simulink model "motion_with_control"  (R2025a)
settings: Solver=FixedStepDiscrete  StartTime=0.0  StopTime=inf  FixedStep=0.01  RelTol=1e-3  EnableMultiTasking=on
PreLoadFcn:
  | frs = FrankaRobotSettings;
libraries: franka_simulink x3
settings Model: SimulationMode=external  ExtModeTrigDuration=10000  Creator=vasi_ko  LastModifiedBy=kvasios
settings SolverCC: ConcurrentTasks=on  AlgebraicLoopSolver=TrustRegion  InsertRTBMode=Never (minimum delay)
settings DataIOCC: LimitDataPoints=on  SaveFormat=Array  ReturnWorkspaceOutputs=off
settings OptimizationCC: DefaultParameterBehavior=Inlined  EnhancedBackFolding=on  PassReuseOutputArgsThreshold=0.0  MaxStackSize=200000  OptimizeBlockOrder=speed  DifferentSizesBufferReuse=on  OptimizationCustomize=off
settings DebuggingCC: SolverPrmCheckMsg=warning  ParameterTunabilityLossMsg=error  UnconnectedInputMsg=warning  UnconnectedOutputMsg=warning  UnconnectedLineMsg=warning  SFUnexpectedBacktrackingDiag=warning  SFNoUnconditionalDefaultTransitionDiag=warning  SFExecutionAtInitializationDiag=none  ArithmeticOperatorsInVariantConditions=warning
settings HardwareCC: ProdBitPerLong=64.0  ProdHWDeviceType=Intel->x86-64 (Linux 64)
settings ModelReferenceCC: EnableRefExpFcnMdlSchedulingChecks=on  PropagateSignalLabelsOutOfModel=off
settings SFSimCC: SimUseLocalCustomCode=off  MATLABDynamicMemAlloc=off  CustomCodeUndefinedFunction=UseInterfaceOnly  SimTargetLang=C++  SimDLTargetLibrary=mkl-dnn
settings RTWCC: HardwareBoard=Generic Linux AMD64 Board  RTWVerbose=off  RTWUseLocalCustomCode=off  BuildConfiguration=Faster Runs  TargetLang=C++  GPUComputeCapability=3.5  DLArmComputeVersion=19.05
settings CodeAppCC: ForceParamTrailComments=on  OperatorAnnotations=on
settings GRTTargetCC: ExtModeStaticAlloc=on  ExtModeMexFile=ext_xcp  ExtModeIntrfLevel=Level2 - Open  MultiInstanceErrorCode=Warning  TargetLangStandard=C++14 (ISO)
settings ConfigComp: CovMetricSettings=dw  CovSaveCumulativeToWorkspaceVar=on  CovSaveSingleToWorkspaceVar=on  CovExternalEMLEnable=off  CovSFcnEnable=off

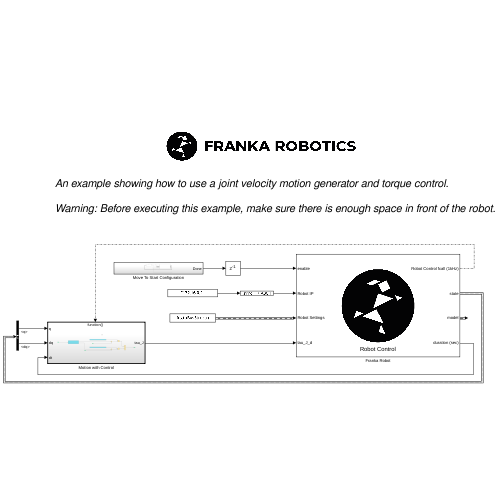
[thumbnail: Simulink's stored preview of the top-level diagram]
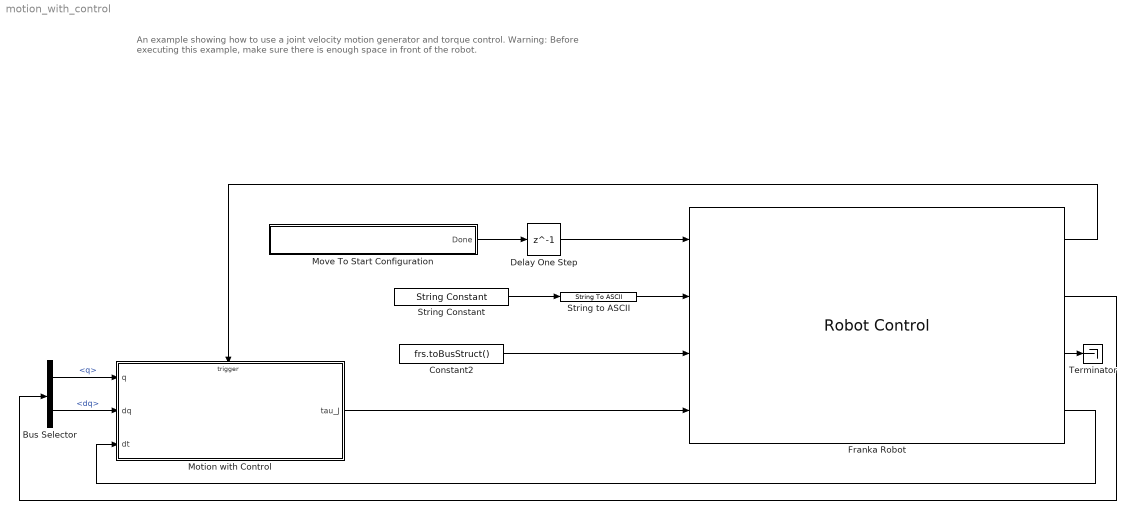
== system motion_with_control ==
  note: An example showing how to use a joint velocity motion generator and torque control.
      |
      | Warning: Before executing this example, make sure there is enough space in front of the robot.
  Bus Selector : BusSelector  OutputSignals=q,dq
  Constant2 : Constant  Value=frs.toBusStruct()  OutDataTypeStr=Bus: FrankaRobotSettingsBus
  Delay One Step : Delay  DelayLength=1
  Franka Robot : franka_simulink/Robot Control  control_mode=Torques
      settings: SourceProductName=Franka Robotics Simulink Support Package
  Motion with Control : Subsystem
      settings: RTWSystemCode=Nonreusable function
  Move To Start Configuration : Subsystem
  String Constant : StringConstant  String="\"172.16.0.2\""
  String to ASCII : StringToASCII  OutputVectorSize=16
  Terminator : Terminator
  wires:
  String to ASCII/1 -> Franka Robot/2
  String Constant/1 -> String to ASCII/1
  Franka Robot/1 -> Motion with Control/Trigger
  Franka Robot/2 -> Bus Selector/1
  Bus Selector/1 -> Motion with Control/1(q)  "<q>"
  Bus Selector/2 -> Motion with Control/2(dq)  "<dq>"
  Franka Robot/4 -> Motion with Control/3(dt)
  Franka Robot/3 -> Terminator/1
  Constant2/1 -> Franka Robot/3
  Motion with Control/1(tau_J) -> Franka Robot/4
  Delay One Step/1 -> Franka Robot/1
  Move To Start Configuration/1(Done) -> Delay One Step/1

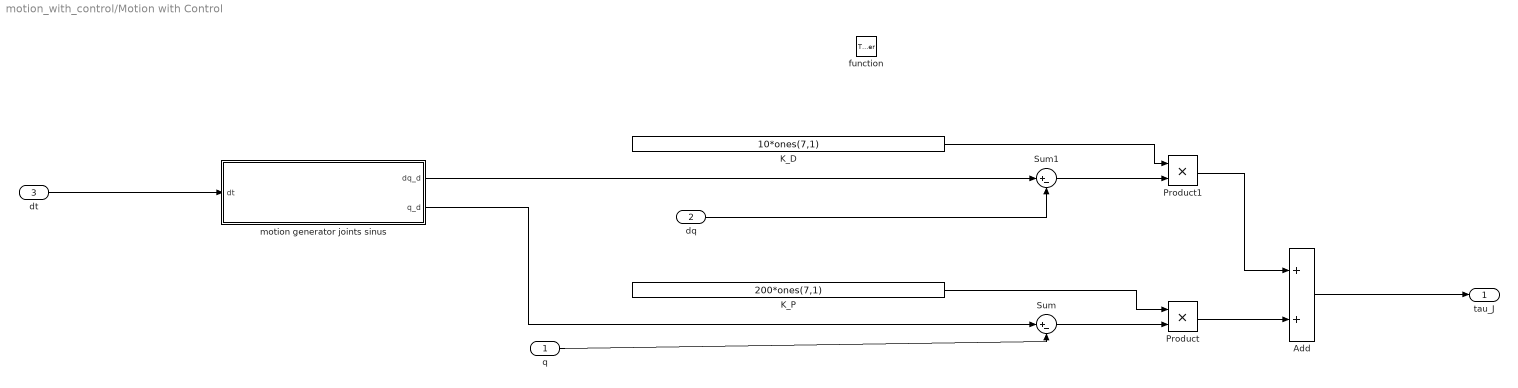
== system motion_with_control/Motion with Control ==
  q : Inport
  dq : Inport  Port=2
  dt : Inport  Port=3
  function : TriggerPort  TriggerType=function-call  VariantControl=(inherit)  SampleTime=0.001
  Add : Sum
  K_D : Constant  Value=10*ones(7,1)  VectorParams1D=off  SampleTime=-1
  K_P : Constant  Value=200*ones(7,1)  VectorParams1D=off  SampleTime=-1
  Product : Product
  Product1 : Product
  Sum : Sum  Inputs=|+-
  Sum1 : Sum  Inputs=|+-
  motion generator joints sinus : Subsystem
      mask Display:
      | pos = get_param(gcb, 'Position');
      | width = pos(3) - pos(1);
      | x = [0:width];
      | y = sin(x/180*pi);
      | % Parameters 'm' and 'b' must be defined in 'Parameters & Dialog' pane.
      | plot(x,y );
      | 
      | port_label('output',1,'dq_d');
      | port_label('output',2,'q_d');
  tau_J : Outport  VectorParamsAs1DForOutWhenUnconnected=off
  wires:
  Product1/1 -> Add/1
  Sum1/1 -> Product1/2
  dq/1 -> Sum1/2
  Product/1 -> Add/2
  Sum/1 -> Product/2
  K_D/1 -> Product1/1
  q/1 -> Sum/2
  K_P/1 -> Product/1
  dt/1 -> motion generator joints sinus/1(dt)
  motion generator joints sinus/1(dq_d) -> Sum1/1
  motion generator joints sinus/2(q_d) -> Sum/1
  Add/1 -> tau_J/1

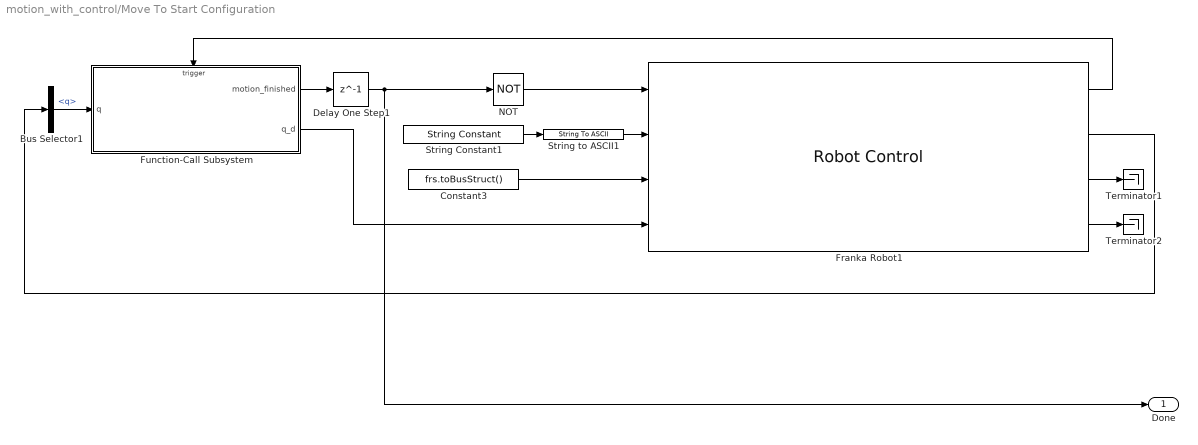
== system motion_with_control/Move To Start Configuration ==
  Bus Selector1 : BusSelector  OutputSignals=q
  Constant3 : Constant  Value=frs.toBusStruct()  OutDataTypeStr=Bus: FrankaRobotSettingsBus
  Delay One Step1 : Delay  DelayLength=1
  Franka Robot1 : franka_simulink/Robot Control  control_mode=Joint Positions
      settings: SourceProductName=Franka Robotics Simulink Support Package
  Function-Call Subsystem : Subsystem  TreatAsAtomicUnit=on
      settings: RTWSystemCode=Nonreusable function
  NOT : Logic  Operator=NOT  IconShape=distinctive  AllPortsSameDT=off  OutDataTypeStr=Inherit: Inherit via back propagation
  String Constant1 : StringConstant  String="\"172.16.0.2\""
  String to ASCII1 : StringToASCII  OutputVectorSize=16
  Terminator1 : Terminator
  Terminator2 : Terminator
  Done : Outport
  wires:
  Function-Call Subsystem/1(motion_finished) -> Delay One Step1/1
  Franka Robot1/1 -> Function-Call Subsystem/Trigger
  Function-Call Subsystem/2(q_d) -> Franka Robot1/4
  String to ASCII1/1 -> Franka Robot1/2
  Delay One Step1/1 -> NOT/1, Done/1
  Constant3/1 -> Franka Robot1/3
  String Constant1/1 -> String to ASCII1/1
  Bus Selector1/1 -> Function-Call Subsystem/1(q)  "<q>"
  Franka Robot1/2 -> Bus Selector1/1
  Franka Robot1/3 -> Terminator1/1
  Franka Robot1/4 -> Terminator2/1
  NOT/1 -> Franka Robot1/1

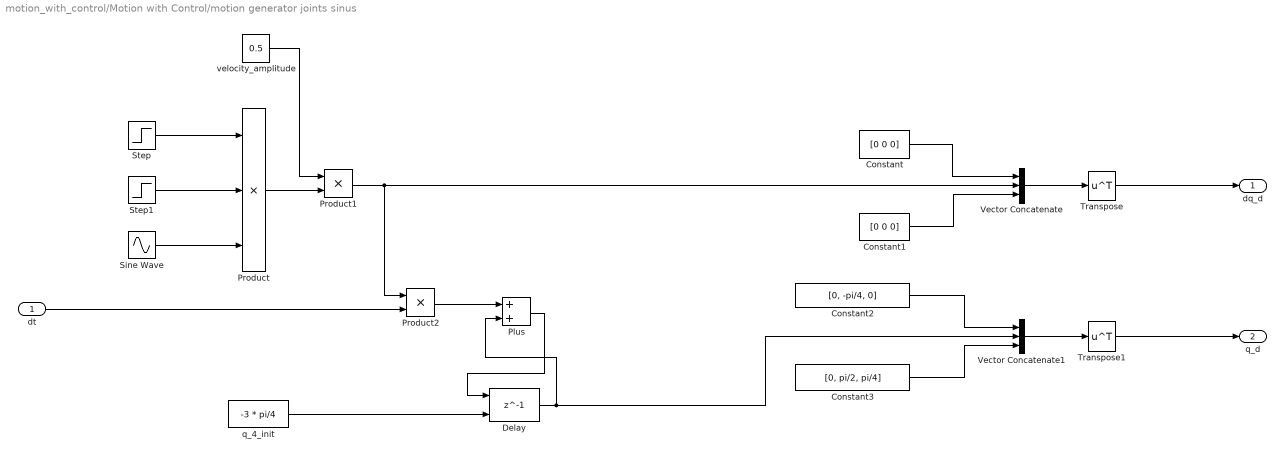
== system motion_with_control/Motion with Control/motion generator joints sinus ==
  dt : Inport
  Constant : Constant  Value=[0 0 0]  VectorParams1D=off
  Constant1 : Constant  Value=[0 0 0]  VectorParams1D=off
  Constant2 : Constant  Value=[0, -pi/4, 0]  VectorParams1D=off
  Constant3 : Constant  Value=[0, pi/2, pi/4]  VectorParams1D=off
  Delay : Delay  DelayLength=1  InitialConditionSource=Input port
      settings: InputPortMap=u0,p4
  Plus : Sum
  Product : Product  Inputs=3
  Product1 : Product
  Product2 : Product
  Sine Wave : Sin  Frequency=pi  Phase=pi
  Step : Step
  Step1 : Step  Time=7  Before=1  After=0
  Transpose : Math  Operator=transpose
  Transpose1 : Math  Operator=transpose
  Vector Concatenate : Concatenate  NumInputs=3
  Vector Concatenate1 : Concatenate  NumInputs=3
  q_4_init : Constant  Value=-3 * pi/4  VectorParams1D=off
  velocity_amplitude : Constant  Value=0.5  VectorParams1D=off
  dq_d : Outport  VectorParamsAs1DForOutWhenUnconnected=off
  q_d : Outport  Port=2  VectorParamsAs1DForOutWhenUnconnected=off
  wires:
  Constant1/1 -> Vector Concatenate/3
  Constant/1 -> Vector Concatenate/1
  Product/1 -> Product1/2
  Sine Wave/1 -> Product/3
  Step/1 -> Product/1
  velocity_amplitude/1 -> Product1/1
  Product1/1 -> Vector Concatenate/2, Product2/1
  Constant3/1 -> Vector Concatenate1/3
  Constant2/1 -> Vector Concatenate1/1
  q_4_init/1 -> Delay/2
  Step1/1 -> Product/2
  dt/1 -> Product2/2
  Delay/1 -> Vector Concatenate1/2, Plus/2
  Plus/1 -> Delay/1
  Product2/1 -> Plus/1
  Vector Concatenate/1 -> Transpose/1
  Vector Concatenate1/1 -> Transpose1/1
  Transpose/1 -> dq_d/1
  Transpose1/1 -> q_d/1

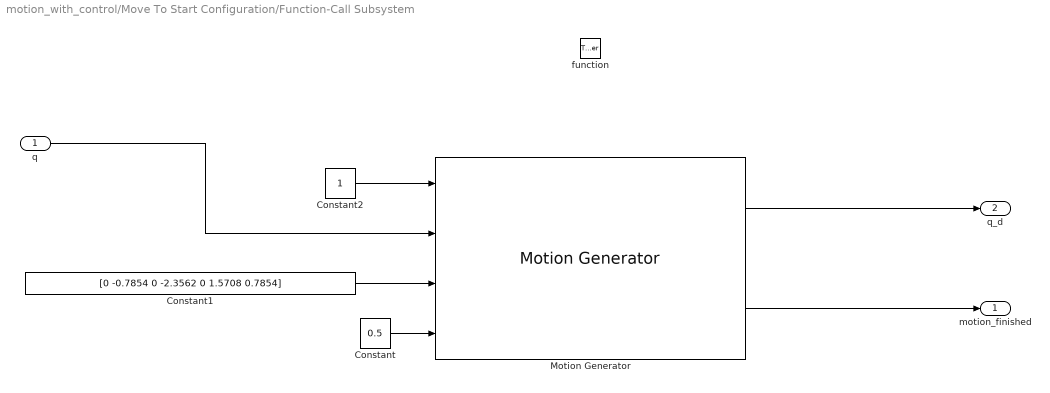
== system motion_with_control/Move To Start Configuration/Function-Call Subsystem ==
  q : Inport
  function : TriggerPort  TriggerType=function-call  VariantControl=(inherit)
  Constant : Constant  Value=0.5
  Constant1 : Constant  Value=[0 -0.7854 0 -2.3562 0 1.5708 0.7854]
  Constant2 : Constant
  Motion Generator : franka_simulink/Motion Generator
      settings: SourceProductName=Franka Robotics Simulink Support Package
  motion_finished : Outport  InitialOutput=0
  q_d : Outport  Port=2  InitialOutput=zeros(7,1)
  wires:
  Motion Generator/1 -> q_d/1
  Constant/1 -> Motion Generator/4
  Constant1/1 -> Motion Generator/3
  q/1 -> Motion Generator/2
  Constant2/1 -> Motion Generator/1
  Motion Generator/2 -> motion_finished/1
